simulink model "DC_model_2"  (R2024a)
settings: Solver=ode3  StartTime=Tstart  StopTime=Tstop  FixedStep=Tsim  RelTol=1e-3  EnableMultiTasking=on
values from neighbouring files (symbols this model uses):
  kth = 0    [DC_model_init.m]
  kw = 0    [DC_model_init.m]
  Ra = 0.075    [DC_model_init.m]    (also in five_bar_init.m)
  Ta = 20e-3    (= 0.02)    [DC_model_init.m]    (also in five_bar_init.m = 0.001)
  Tm = 0.5    [DC_model_init.m]    (also in five_bar_init.m)
  Tsim = 10e-3    (= 0.01)    [DC_model_init.m]    (also in five_bar_init.m = 0.001)
  Tth = 1    [DC_model_init.m]
  Up = (1-Ra)    (= 0.925)    [DC_model_init.m]
libraries: slpidlib x2
settings Model: Creator=Pop
settings SolverCC: AlgebraicLoopSolver=TrustRegion
settings DataIOCC: LimitDataPoints=on  SaveFormat=Array  ReturnWorkspaceOutputs=off
settings OptimizationCC: LifeSpan=inf
settings DebuggingCC: SolverPrmCheckMsg=warning  UnconnectedInputMsg=warning  UnconnectedOutputMsg=warning  UnconnectedLineMsg=warning  SFUnexpectedBacktrackingDiag=warning  SFNoUnconditionalDefaultTransitionDiag=warning  SFExecutionAtInitializationDiag=none  ArithmeticOperatorsInVariantConditions=warning
settings HardwareCC: ProdBitPerPointer=32  ProdBitPerSizeT=32  ProdBitPerPtrDiffT=32  ProdLargestAtomicFloat=None  ProdIntDivRoundTo=Undefined  ProdEndianess=Unspecified  ProdWordSize=32  ProdHWDeviceType=32-bit Generic
settings ModelReferenceCC: PropagateSignalLabelsOutOfModel=off
settings SFSimCC: SimUseLocalCustomCode=off  CustomCodeUndefinedFunction=UseInterfaceOnly
settings RTWCC: RTWUseLocalCustomCode=off  GPUComputeCapability=3.5
settings CodeAppCC: StateflowObjectComments=on
settings GRTTargetCC: TargetLangStandard=C89/C90 (ANSI)
settings ConfigComp: CovMetricSettings=dw  CovSaveCumulativeToWorkspaceVar=on  CovSaveSingleToWorkspaceVar=on  CovExternalEMLEnable=off  CovSFcnEnable=off

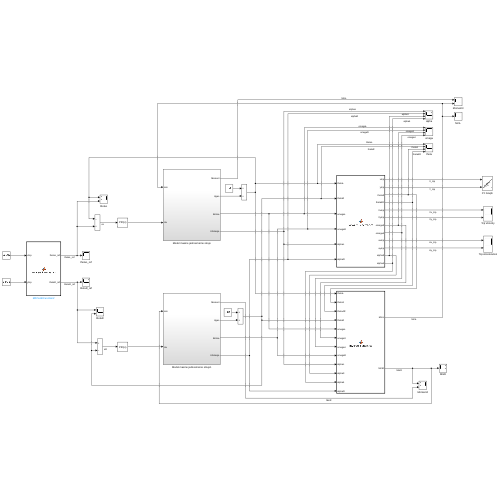
[thumbnail: Simulink's stored preview of the top-level diagram]
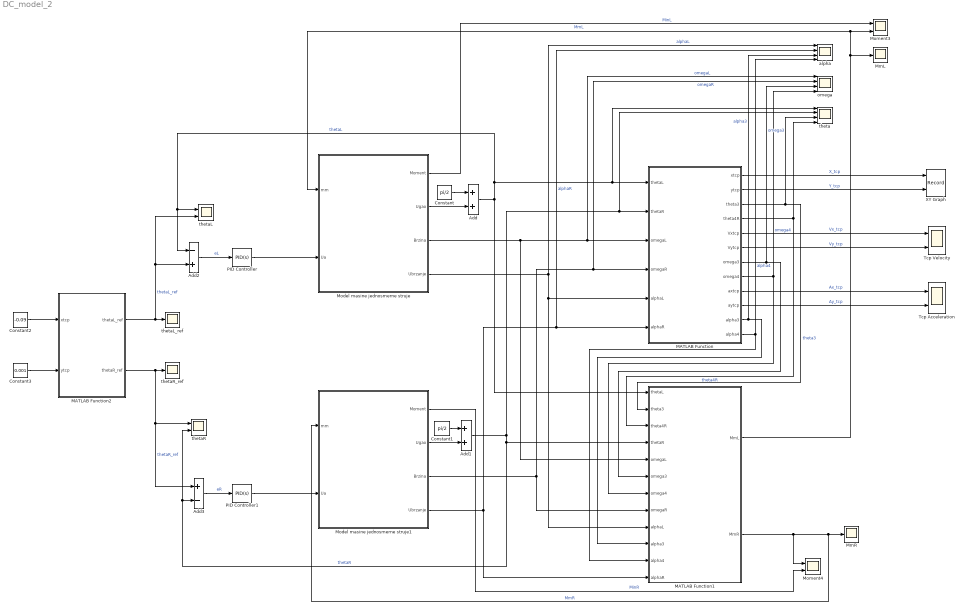
== system DC_model_2 ==
  Add : Sum
  Add1 : Sum
  Add2 : Sum  Inputs=-+
  Add3 : Sum  Inputs=+-
  Constant : Constant  Value=pi/2
  Constant1 : Constant  Value=pi/2
  Constant2 : Constant  Value=-0.09
  Constant3 : Constant  Value=0.001
  MATLAB Function : MATLAB Function  TreatAsAtomicUnit=on
  MATLAB Function1 : MATLAB Function  TreatAsAtomicUnit=on
  MATLAB Function2 : MATLAB Function  TreatAsAtomicUnit=on
  MmL : Scope
  MmR : Scope
  Model masine jednosmerne struje : Subsystem
  Model masine jednosmerne struje1 : Subsystem
  Moment3 : Scope  NumInputPorts=2
  Moment4 : Scope  NumInputPorts=2
  PID Controller : slpidlib/PID Controller  Controller=PID  Form=Parallel  TimeDomain=Continuous-time  UseExternalTs=off  SampleTime=-1  IntegratorMethod=Forward Euler  FilterMethod=Forward Euler  ControllerParametersSource=internal  P=1  I=0  UseKiTs=off  D=0  UseExternalDerivativeSource=off  N=100  UseFilter=on  TunerSelectOption=Transfer Function Based (PID Tuner App)  InitialConditionSource=internal  InitialConditionForIntegrator=0  InitialConditionForFilter=0  DifferentiatorICPrevScaledInput=0  ExternalReset=none  TrackingMode=off  Kt=1  LimitOutput=off  SatLimitsSource=internal  UpperSaturationLimit=inf  LowerSaturationLimit=-inf  LinearizeAsGain=on  AntiWindupMode=none  Kb=1  LimitIntegrator=off  UpperIntegratorSaturationLimit=inf  LowerIntegratorSaturationLimit=-inf  POutMin=[]  POutMax=[]  IOutMin=[]  IOutMax=[]  DOutMin=[]  DOutMax=[]  NOutMin=[]  NOutMax=[]  SumOutMin=[]  SumOutMax=[]  SaturationOutMin=[]  SaturationOutMax=[]  PParamMin=[]  PParamMax=[]  IParamMin=[]  IParamMax=[]  DParamMin=[]  DParamMax=[]  NParamMin=[]  NParamMax=[]  KbParamMin=[]  KbParamMax=[]  KtParamMin=[]  KtParamMax=[]  KbOutMin=[]  KbOutMax=[]  KtOutMin=[]  KtOutMax=[]  IntegratorOutMin=[]  IntegratorOutMax=[]  FilterOutMin=[]  FilterOutMax=[]  SumI1OutMin=[]  SumI1OutMax=[]  SumI2OutMin=[]  SumI2OutMax=[]  SumI3OutMin=[]  SumI3OutMax=[]  SumI4OutMin=[]  SumI4OutMax=[]  SumDOutMin=[]  SumDOutMax=[]  DifferentiatorOutMin=[]  DifferentiatorOutMax=[]  FilterDiffOutCoefMin=[]  FilterDiffOutCoefMax=[]  ReciprocalOutMin=[]  ReciprocalOutMax=[]  SumDenOutMin=[]  SumDenOutMax=[]  SumNumOutMin=[]  SumNumOutMax=[]  DivideOutMin=[]  DivideOutMax=[]  UdiffTsProdOutMin=[]  UdiffTsProdOutMax=[]  NTsProdOutMin=[]  NTsProdOutMax=[]  UintegralTsProdOutMin=[]  UintegralTsProdOutMax=[]  UngainTsProdOutMin=[]  UngainTsProdOutMax=[]  ClampingZeroOutDataTypeStr=Inherit: Inherit via back propagation  ClampingZeroOutMin=[]  ClampingZeroOutMax=[]  FilterDenConstantOutDataTypeStr=Inherit: Inherit via back propagation  FilterDenConstantOutMin=[]  FilterDenConstantOutMax=[]  PCopyOutDataTypeStr=Inherit: Inherit via back propagation  PCopyOutMin=[]  PCopyOutMax=[]  NCopyOutDataTypeStr=Inherit: Inherit via back propagation  NCopyOutMin=[]  NCopyOutMax=[]  IntegratorContinuousStateAttributes=''  IntegratorStateMustResolveToSignalObject=off  IntegratorRTWStateStorageClass=Auto  FilterContinuousStateAttributes=''  FilterStateMustResolveToSignalObject=off  FilterRTWStateStorageClass=Auto  ParallelPVariant=InternalParameters  IdealPVariant=Disabled  IVariant=InternalParameters  DVariant=InternalParameters  IntegratorVariant=Continuous  SatVariant=Disabled  AWVariant=Passthrough  PCopyVariant=Disabled  TRVariant=Disabled  FdbkBlocksVariant=Forward  IdealPFdbkVariant=Disabled  SatFdbkVariant=Disabled  DerivativeFilterVariant=ContFilter  NVariant=InternalParameters  NCopyVariant=Disabled  FilterICVariant=InternalICsFilter  IntegratorICVariant=InternalICs  ExternalResetVariant=Disabled  TRSumVariant=Passthrough  SumFdbkVariant=Disabled  SumVariant=Sum_PID  TsampFilterVariant=InternalTs  TsampNgainVariant=Passthrough  TsampIntegralVariant=Disabled_SignalSpec  ExternalSaturationOutDataTypeStr=Inherit: Same as second input  DerivativeSourceVariant=ErrorSignal
  PID Controller1 : slpidlib/PID Controller  Controller=PID  Form=Parallel  TimeDomain=Continuous-time  UseExternalTs=off  SampleTime=-1  IntegratorMethod=Forward Euler  FilterMethod=Forward Euler  ControllerParametersSource=internal  P=1  I=0  UseKiTs=off  D=0  UseExternalDerivativeSource=off  N=100  UseFilter=on  TunerSelectOption=Transfer Function Based (PID Tuner App)  InitialConditionSource=internal  InitialConditionForIntegrator=0  InitialConditionForFilter=0  DifferentiatorICPrevScaledInput=0  ExternalReset=none  TrackingMode=off  Kt=1  LimitOutput=off  SatLimitsSource=internal  UpperSaturationLimit=inf  LowerSaturationLimit=-inf  LinearizeAsGain=on  AntiWindupMode=none  Kb=1  LimitIntegrator=off  UpperIntegratorSaturationLimit=inf  LowerIntegratorSaturationLimit=-inf  POutMin=[]  POutMax=[]  IOutMin=[]  IOutMax=[]  DOutMin=[]  DOutMax=[]  NOutMin=[]  NOutMax=[]  SumOutMin=[]  SumOutMax=[]  SaturationOutMin=[]  SaturationOutMax=[]  PParamMin=[]  PParamMax=[]  IParamMin=[]  IParamMax=[]  DParamMin=[]  DParamMax=[]  NParamMin=[]  NParamMax=[]  KbParamMin=[]  KbParamMax=[]  KtParamMin=[]  KtParamMax=[]  KbOutMin=[]  KbOutMax=[]  KtOutMin=[]  KtOutMax=[]  IntegratorOutMin=[]  IntegratorOutMax=[]  FilterOutMin=[]  FilterOutMax=[]  SumI1OutMin=[]  SumI1OutMax=[]  SumI2OutMin=[]  SumI2OutMax=[]  SumI3OutMin=[]  SumI3OutMax=[]  SumI4OutMin=[]  SumI4OutMax=[]  SumDOutMin=[]  SumDOutMax=[]  DifferentiatorOutMin=[]  DifferentiatorOutMax=[]  FilterDiffOutCoefMin=[]  FilterDiffOutCoefMax=[]  ReciprocalOutMin=[]  ReciprocalOutMax=[]  SumDenOutMin=[]  SumDenOutMax=[]  SumNumOutMin=[]  SumNumOutMax=[]  DivideOutMin=[]  DivideOutMax=[]  UdiffTsProdOutMin=[]  UdiffTsProdOutMax=[]  NTsProdOutMin=[]  NTsProdOutMax=[]  UintegralTsProdOutMin=[]  UintegralTsProdOutMax=[]  UngainTsProdOutMin=[]  UngainTsProdOutMax=[]  ClampingZeroOutDataTypeStr=Inherit: Inherit via back propagation  ClampingZeroOutMin=[]  ClampingZeroOutMax=[]  FilterDenConstantOutDataTypeStr=Inherit: Inherit via back propagation  FilterDenConstantOutMin=[]  FilterDenConstantOutMax=[]  PCopyOutDataTypeStr=Inherit: Inherit via back propagation  PCopyOutMin=[]  PCopyOutMax=[]  NCopyOutDataTypeStr=Inherit: Inherit via back propagation  NCopyOutMin=[]  NCopyOutMax=[]  IntegratorContinuousStateAttributes=''  IntegratorStateMustResolveToSignalObject=off  IntegratorRTWStateStorageClass=Auto  FilterContinuousStateAttributes=''  FilterStateMustResolveToSignalObject=off  FilterRTWStateStorageClass=Auto  ParallelPVariant=InternalParameters  IdealPVariant=Disabled  IVariant=InternalParameters  DVariant=InternalParameters  IntegratorVariant=Continuous  SatVariant=Disabled  AWVariant=Passthrough  PCopyVariant=Disabled  TRVariant=Disabled  FdbkBlocksVariant=Forward  IdealPFdbkVariant=Disabled  SatFdbkVariant=Disabled  DerivativeFilterVariant=ContFilter  NVariant=InternalParameters  NCopyVariant=Disabled  FilterICVariant=InternalICsFilter  IntegratorICVariant=InternalICs  ExternalResetVariant=Disabled  TRSumVariant=Passthrough  SumFdbkVariant=Disabled  SumVariant=Sum_PID  TsampFilterVariant=InternalTs  TsampNgainVariant=Passthrough  TsampIntegralVariant=Disabled_SignalSpec  ExternalSaturationOutDataTypeStr=Inherit: Same as second input  DerivativeSourceVariant=ErrorSignal
  Tcp Acceleration : Scope  NumInputPorts=2
  Tcp Velocity : Scope  NumInputPorts=2
  XY Graph : Record  FileSettingsInternal="{\"entries\":[{\"content\":{\"excelSettings\":{\"content\":{},\"type\":\"Streamout.ExcelSettings\"}},\"type\":\"Streamout.FileSettingStorage\",\"uuid\":\"\"}],\"packageUris\":[\"http:\\/\\/schema.mathworks.com\\/mf0\\/streamout_blocks\\/R2020a\"],\"version\":\"1.0\"}"  Layout=[1 1]  SignalsInternal="{\"entries\":[{\"content\":{\"signals\":[{\"content\":{\"blockPath\":[],\"dimensions\":[1],\"domain\":\"\",\"lineColor\":\"#a2142f\",\"plots\":[ 1 ],\"port\":1,\"sid\":[\"\"],\"signalID\":1,\"signalName\":\"X_tcp\"},\"type\":\"RecordBlkView.Signal\",\"uuid\":\"\"},{\"content\":{\"blockPath\":[],\"dimensions\":[1],\"domain\":\"\",\"lineColor\":\"#139fff\",\"plots\":[ 1 ],\"port\":2,\"sid\":[\"\"],\"signalID\":2,\"signalName\":\"Y_tcp\"},\"type\":\"RecordBlkView.Signal\",\"uuid\":\"\"}]},\"type\":\"RecordBlkView.InputSignals\",\"uuid\":\"\"}],\"packageUris\":[\"http:\\/\\/schema.mathworks.com\\/mf0\\/streamout_blocks\\/R2020a\"],\"version\":\"1.0\"}"  VisualizationBindings="{\"xyplotplugin\":{\"info\":[{\"series\":[{\"bindingParametersList\":[{\"parameter\":\"X-Axis\",\"signalID\":1,\"signalName\":\"X_tcp\"},{\"parameter\":\"Y-Axis\",\"signalID\":2,\"signalName\":\"Y_tcp\"}],\"seriesID\":0}],\"subplotID\":1}]}}"  CompatibilityTag=XY
  alpha : Scope  NumInputPorts=4
  omega : Scope  NumInputPorts=4
  theta : Scope  NumInputPorts=4
  thetaL : Scope  NumInputPorts=2
  thetaL_ref : Scope
  thetaR : Scope  NumInputPorts=2
  thetaR_ref : Scope
  wires:
  Model masine jednosmerne struje/1(Moment) -> Moment3/1  "MinL"
  MATLAB Function/1(xtcp) -> XY Graph/1  "X_tcp"
  MATLAB Function/2(ytcp) -> XY Graph/2  "Y_tcp"
  MATLAB Function1/1(MmL) -> Model masine jednosmerne struje/1(mm), Moment3/2, MmL/1  "MmL"
  MATLAB Function1/2(MmR) -> Model masine jednosmerne struje1/1(mm), MmR/1, Moment4/1  "MmR"
  Model masine jednosmerne struje1/1(Moment) -> Moment4/2  "MinR"
  Add/1 -> thetaL/1, Add2/1, theta/1, MATLAB Function/1(thetaL), MATLAB Function1/1(thetaL)  "thetaL"
  Add1/1 -> thetaR/2, Add3/2, MATLAB Function1/4(thetaR), theta/2, MATLAB Function/2(thetaR)  "thetaR"
  Model masine jednosmerne struje/3(Brzina) -> MATLAB Function1/5(omegaL), omega/1, MATLAB Function/3(omegaL)  "omegaL"
  Model masine jednosmerne struje1/3(Brzina) -> omega/2, MATLAB Function/4(omegaR), MATLAB Function1/8(omegaR)  "omegaR"
  Model masine jednosmerne struje/4(Ubrzanje) -> MATLAB Function/5(alphaL), MATLAB Function1/9(alphaL), alpha/1  "alphaL"
  Model masine jednosmerne struje1/4(Ubrzanje) -> MATLAB Function1/12(alphaR), MATLAB Function/6(alphaR), alpha/2  "alphaR"
  MATLAB Function/3(theta3) -> theta/3, MATLAB Function1/2(theta3)  "theta3"
  MATLAB Function/4(theta4R) -> theta/4, MATLAB Function1/3(theta4R)  "theta4R"
  MATLAB Function/7(omega3) -> omega/3, MATLAB Function1/6(omega3)  "omega3"
  MATLAB Function/8(omega4) -> omega/4, MATLAB Function1/7(omega4)  "omega4"
  MATLAB Function/11(alpha3) -> alpha/3, MATLAB Function1/10(alpha3)  "alpha3"
  MATLAB Function/12(alpha4) -> alpha/4, MATLAB Function1/11(alpha4)  "alpha4"
  MATLAB Function/5(Vxtcp) -> Tcp Velocity/1  "Vx_tcp"
  MATLAB Function/6(Vytcp) -> Tcp Velocity/2  "Vy_tcp"
  MATLAB Function/9(axtcp) -> Tcp Acceleration/1  "Ax_tcp"
  MATLAB Function/10(aytcp) -> Tcp Acceleration/2  "Ay_tcp"
  Model masine jednosmerne struje/2(Ugao) -> Add/2
  Constant/1 -> Add/1
  Constant1/1 -> Add1/1
  Model masine jednosmerne struje1/2(Ugao) -> Add1/2
  Constant2/1 -> MATLAB Function2/1(xtcp)
  Constant3/1 -> MATLAB Function2/2(ytcp)
  MATLAB Function2/1(thetaL_ref) -> thetaL/2, Add2/2, thetaL_ref/1  "thetaL_ref"
  MATLAB Function2/2(thetaR_ref) -> thetaR/1, Add3/1, thetaR_ref/1  "thetaR_ref"
  Add2/1 -> PID Controller/1  "eL"
  Add3/1 -> PID Controller1/1  "eR"
  PID Controller/1 -> Model masine jednosmerne struje/2(Ua)
  PID Controller1/1 -> Model masine jednosmerne struje1/2(Ua)

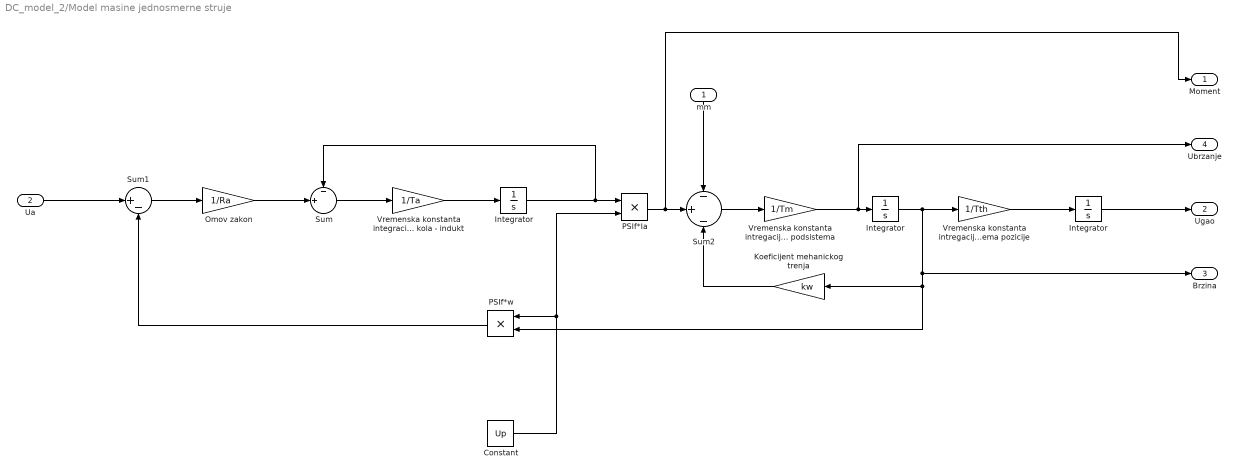
== system DC_model_2/Model masine jednosmerne struje ==
  mm : Inport
  Ua : Inport  Port=2
  "   Integrator   " : Integrator
  "  Integrator  " : Integrator
  Constant : Constant  Value=Up
  Integrator : Integrator
  Koeficijent mehanickog trenja : Gain  Gain=kw  SampleTime=Tsim
  Omov zakon : Gain  Gain=1/Ra  SampleTime=Tsim
  PSIf*Ia : Product  SampleTime=Tsim
  PSIf*w : Product  SampleTime=Tsim
  Sum : Sum  Inputs=-|+||  SampleTime=Tsim
  Sum1 : Sum  Inputs=|+-  SampleTime=Tsim
  Sum2 : Sum  Inputs=-||+||-  SampleTime=Tsim
  Vremenska konstanta integracije rotorskog kola - indukt : Gain  Gain=1/Ta  SampleTime=Tsim
  Vremenska konstanta intregacije mehanickog podsistema : Gain  Gain=1/Tm  SampleTime=Tsim
  Vremenska konstanta intregacije podsistema pozicije : Gain  Gain=1/Tth  SampleTime=Tsim
  Moment : Outport
  Ugao : Outport  Port=2
  Brzina : Outport  Port=3
  Ubrzanje : Outport  Port=4
  wires:
  Omov zakon/1 -> Sum/2
  Sum1/1 -> Omov zakon/1
  Integrator/1 -> Sum/1, PSIf*Ia/1
  Sum/1 -> Vremenska konstanta integracije rotorskog kola - indukt/1
  Vremenska konstanta integracije rotorskog kola - indukt/1 -> Integrator/1
  PSIf*Ia/1 -> Moment/1, Sum2/2
  Sum2/1 -> Vremenska konstanta intregacije mehanickog podsistema/1
  Vremenska konstanta intregacije mehanickog podsistema/1 -> Ubrzanje/1, "  Integrator  "/1
  Koeficijent mehanickog trenja/1 -> Sum2/3
  Vremenska konstanta intregacije podsistema pozicije/1 -> "   Integrator   "/1
  mm/1 -> Sum2/1
  Constant/1 -> PSIf*w/1, PSIf*Ia/2
  PSIf*w/1 -> Sum1/2
  "   Integrator   "/1 -> Ugao/1
  "  Integrator  "/1 -> Vremenska konstanta intregacije podsistema pozicije/1, PSIf*w/2, Koeficijent mehanickog trenja/1, Brzina/1
  Ua/1 -> Sum1/1

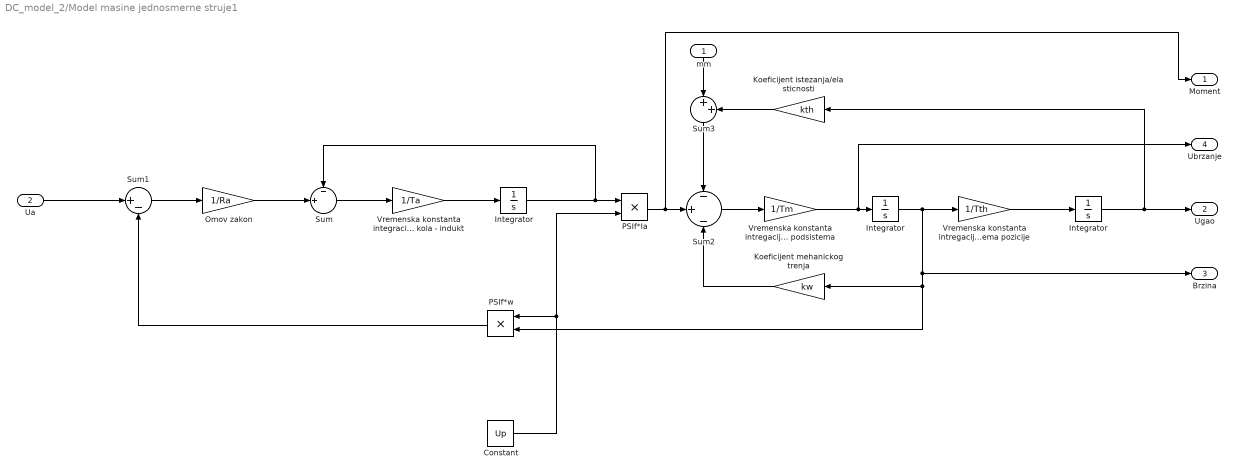
== system DC_model_2/Model masine jednosmerne struje1 ==
  mm : Inport
  Ua : Inport  Port=2
  "   Integrator   " : Integrator
  "  Integrator  " : Integrator
  Constant : Constant  Value=Up
  Integrator : Integrator
  Koeficijent istezanja/elasticnosti : Gain  Gain=kth  SampleTime=Tsim
  Koeficijent mehanickog trenja : Gain  Gain=kw  SampleTime=Tsim
  Omov zakon : Gain  Gain=1/Ra  SampleTime=Tsim
  PSIf*Ia : Product  SampleTime=Tsim
  PSIf*w : Product  SampleTime=Tsim
  Sum : Sum  Inputs=-|+||  SampleTime=Tsim
  Sum1 : Sum  Inputs=|+-  SampleTime=Tsim
  Sum2 : Sum  Inputs=-||+||-  SampleTime=Tsim
  Sum3 : Sum  Inputs=|++  SampleTime=Tsim
  Vremenska konstanta integracije rotorskog kola - indukt : Gain  Gain=1/Ta  SampleTime=Tsim
  Vremenska konstanta intregacije mehanickog podsistema : Gain  Gain=1/Tm  SampleTime=Tsim
  Vremenska konstanta intregacije podsistema pozicije : Gain  Gain=1/Tth  SampleTime=Tsim
  Moment : Outport
  Ugao : Outport  Port=2
  Brzina : Outport  Port=3
  Ubrzanje : Outport  Port=4
  wires:
  Omov zakon/1 -> Sum/2
  Sum1/1 -> Omov zakon/1
  Integrator/1 -> Sum/1, PSIf*Ia/1
  Sum/1 -> Vremenska konstanta integracije rotorskog kola - indukt/1
  Vremenska konstanta integracije rotorskog kola - indukt/1 -> Integrator/1
  PSIf*Ia/1 -> Moment/1, Sum2/2
  Sum2/1 -> Vremenska konstanta intregacije mehanickog podsistema/1
  Vremenska konstanta intregacije mehanickog podsistema/1 -> Ubrzanje/1, "  Integrator  "/1
  Koeficijent mehanickog trenja/1 -> Sum2/3
  Vremenska konstanta intregacije podsistema pozicije/1 -> "   Integrator   "/1
  Sum3/1 -> Sum2/1
  Koeficijent istezanja/elasticnosti/1 -> Sum3/2
  Constant/1 -> PSIf*w/1, PSIf*Ia/2
  PSIf*w/1 -> Sum1/2
  "   Integrator   "/1 -> Koeficijent istezanja/elasticnosti/1, Ugao/1
  "  Integrator  "/1 -> Vremenska konstanta intregacije podsistema pozicije/1, PSIf*w/2, Koeficijent mehanickog trenja/1, Brzina/1
  Ua/1 -> Sum1/1
  mm/1 -> Sum3/1

== matlab function DC_model_2/MATLAB Function1 ==
  data: thetaL input; MmL output; theta3 input; theta4R input; thetaR input; omegaL input; omega3 input; omega4 input; omegaR input; alphaL input; alpha3 input; alpha4 input; alphaR input; MmR output
function [MmL, MmR] = inverse_dynamics(thetaL, theta3, theta4R, thetaR, omegaL, omega3, omega4, omegaR, alphaL, alpha3, alpha4, alphaR)
    [~, P, D, mP, mD, JsP, JsD] = get_params();
    
    m2 = mP;
    m5 = mP;
    m3 = mD;
    m4 = mD;
    Js2 = JsP;
    Js5 = JsP;
    Js3 = JsD;
    Js4 = JsD;
    
    as2x = - P/2 * omegaL^2 * cos(thetaL) - P/2 * alphaL * sin(thetaL);
    as2y = - P/2 * omegaL^2 * sin(thetaL) + P/2 * alphaL * cos(thetaL);
    as3x = - P * omegaL^2 * cos(thetaL) - P * alphaL * sin(thetaL) - D/2 * omega3^2 * cos(theta3) - D/2 * alpha3 * sin(theta3);
    as3y = - P * omegaL^2 * sin(thetaL) + P * alphaL * cos(thetaL) - D/2 * omega3^2 * sin(theta3) + D/2 * alpha3 * cos(theta3);
    as4x = - P * omegaR^2 * cos(thetaR) - P * alphaR * sin(thetaR) - D/2 * omega4^2 * cos(theta4R) - D/2 * alpha4 * sin(theta4R);
    as4y = - P * omegaR^2 * sin(thetaR) + P * alphaR * cos(thetaR) - D/2 * omega4^2 * sin(theta4R) + D/2 * alpha4 * cos(theta4R);
    as5x = - P/2 * omegaR^2 * cos(thetaR) - P/2 * alphaR * sin(thetaR);
    as5y = - P/2 * omegaR^2 * sin(thetaR) + P/2 * alphaR * cos(thetaR);

    A_d = [ 1, 0, 0, 1, 0, 0, 0, 0, 0, 0, 0, 0;
            0, 1, 0, 0, 1, 0, 0, 0, 0, 0, 0, 0;
            P/2*sin(thetaL), -P/2*cos(thetaL), 1, -P/2*sin(thetaL), P/2*cos(thetaL), 0, 0, 0, 0, 0, 0, 0;
            0, 0, 0, -1, 0, 1, 0, 0, 0, 0, 0, 0;
            0, 0, 0, 0, -1, 0, 1, 0, 0, 0, 0, 0;
            0, 0, 0, -D/2*sin(theta3), D/2*cos(theta3), -D/2*sin(theta3), D/2*cos(theta3), 0, 0, 0, 0, 0;
            0, 0, 0, 0, 0, -1, 0, 1, 0, 0, 0, 0;
            0, 0, 0, 0, 0, 0, -1, 0, 1, 0, 0, 0;
            0, 0, 0, 0, 0, D/2*sin(theta4R), -D/2*cos(theta4R), D/2*sin(theta4R), -D/2*cos(theta4R), 0, 0, 0;
            0, 0, 0, 0, 0, 0, 0, -1, 0, 1, 0, 0;
            0, 0, 0, 0, 0, 0, 0, 0, -1, 0, 1, 0;
            0, 0, 0, 0, 0, 0, 0, -P/2*sin(thetaR), P/2*cos(thetaR), -P/2*sin(thetaR), P/2*cos(thetaR), 1
          ];
    B_d = [ m2 * as2x;
            m2 * as2y;
            Js2 * alphaL;
            m3 * as3x;
            m3 * as3y;
            Js3 * alpha3;
            m4 * as4x;
            m4 * as4y;
            Js4 * alpha4;
            m5 * as5x;
            m5 * as5y;
            Js5 * alphaR
          ];
    D = A_d \ B_d;
    MmL = D(3);
    MmR = D(12);
end

== matlab function DC_model_2/MATLAB Function ==
  data: thetaL input; xtcp output; thetaR input; omegaL input; omegaR input; alphaL input; alphaR input; ytcp output; theta3 output; theta4R output; Vxtcp output; Vytcp output; omega3 output; omega4 output; axtcp output; aytcp output; alpha3 output; alpha4 output
function [xtcp, ytcp, theta3, theta4R, Vxtcp, Vytcp, omega3, omega4, axtcp, aytcp, alpha3, alpha4] = forward_kinematics(thetaL, thetaR, omegaL, omegaR, alphaL, alphaR)
    [L,P,D] = get_params();

    xA = -L/2 + P * cos(thetaL);
    yA = P * sin(thetaL);
    xB = L/2 + P * cos(thetaR);
    yB = P * sin(thetaR);

    A = (xB - xA) / D;
    B = (yB - yA) / D;
    C = (A*A + B*B) / 2;
    A1 = (xA - xB) / D;
    B1 = (yA - yB) / D;

    theta4R = 2*atan2(-B-sqrt(A*A+B*B-C*C), C-A);
    theta3 = 2*atan2(-B1+sqrt(A1*A1+B1*B1-C*C), C-A1);
    xtcp = xA + D*cos(theta3);
    ytcp = yA + D*sin(theta3);

    % Velocities
    A_v = [ -1/(P*sin(thetaL)), 0, - D*sin(theta3)/(P*sin(thetaL)), 0;
            -1/(P*sin(thetaR)), 0, 0, - D*sin(theta4R)/(P*sin(thetaR));
            0, 1/(P*cos(thetaL)), - D*cos(theta3)/(P*cos(thetaL)), 0;
            0, 1/(P*cos(thetaR)), 0, - D*cos(theta4R)/(P*cos(thetaR))
            ];
    B_v = [ omegaL;
            omegaR;
            omegaL;
            omegaR
          ];
    V = A_v \ B_v;
    Vxtcp = V(1);
    Vytcp = V(2);
    omega3 = V(3);
    omega4 = V(4);

    % Accelerations
    A_a = [ 1, 0, D*sin(theta3), 0;
            1, 0, 0, D*sin(theta4R);
            0, 1, -D*cos(theta3), 0;
            0, 1, 0, -D*cos(theta4R)
            ];
    B_a = [ -P*sin(thetaL)*alphaL - P*cos(thetaL)*omegaL^2 - D*cos(theta3)*omega3^2;
            -P*sin(thetaR)*alphaR - P*cos(thetaR)*omegaR^2 - D*cos(theta4R)*omega4^2;
            P*cos(thetaL)*alphaL - P*sin(thetaL)*omegaL^2 - D*sin(theta3)*omega3^2;
            P*cos(thetaR)*alphaR - P*sin(thetaR)*omegaR^2 - D*sin(theta4R)*omega4^2
          ];
    A = A_a \ B_a;
    axtcp = A(1);
    aytcp = A(2);
    alpha3 = A(3);
    alpha4 = A(4);
end

== matlab function DC_model_2/MATLAB Function2 ==
  data: xtcp input; thetaL_ref output; ytcp input; thetaR_ref output
function [thetaL_ref, thetaR_ref] = inverse_kinematics(xtcp,ytcp)
    [L,P,D] = get_params();

    C1 = ((xtcp + L/2)^2 + ytcp^2 + P^2 - D^2) / (2*ytcp*P);
    C2 = (xtcp + L/2) / ytcp;
    C3 = ((xtcp - L/2)^2 + ytcp^2 + P^2 - D^2) / (2*ytcp*P);
    C4 = (xtcp - L/2) / ytcp;

    thetaL_ref = 2*atan2(1+sqrt(1-C1*C1+C2*C2), C1+C2);
    thetaR_ref = 2*atan2(1-sqrt(1-C3*C3+C4*C4), C3+C4);

    thetaL_ref = wrapTo2Pi(thetaL_ref);
    thetaR_ref = wrapToPi(thetaR_ref);
end
